simulink model "DCPF_WithDroopCPL"  (R2015b)
settings: Solver=VariableStepAuto  StartTime=0.0  StopTime=1.0  RelTol=1e-3
undefined symbols (not defined in the file or in its folder): C_dc_link, V_dc_link_initial
libraries: powerlib x21
settings Model: Creator=Irina  LastModifiedBy=Irina

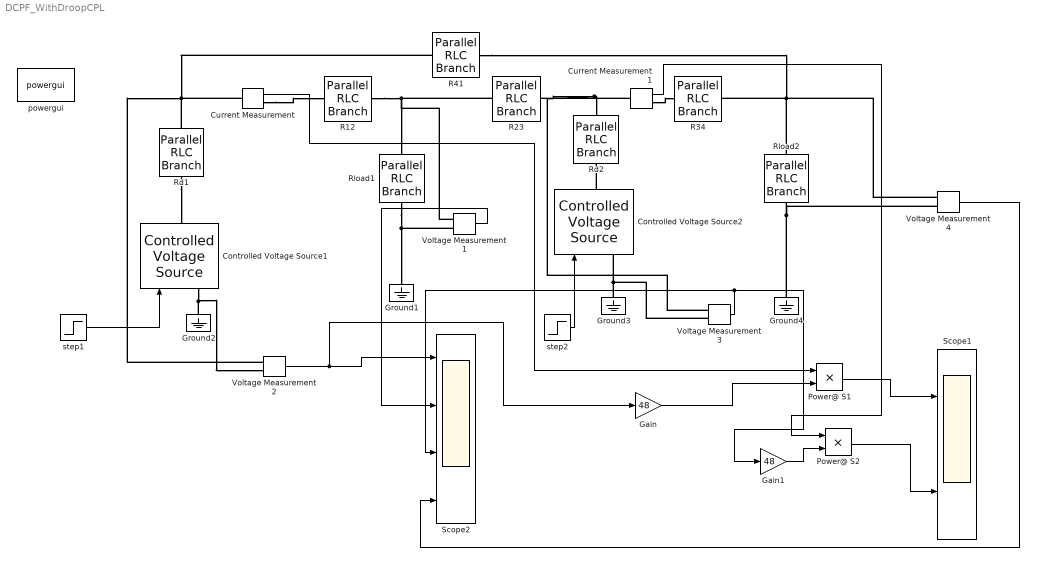
== system DCPF_WithDroopCPL ==
  Controlled Voltage Source1 : powerlib/Electrical Sources/Controlled Voltage Source  Initialize=on  Source_Type=DC  Amplitude=48  Phase=0  Frequency=0  Measurements=None
  Controlled Voltage Source2 : powerlib/Electrical Sources/Controlled Voltage Source  Initialize=on  Source_Type=DC  Amplitude=48  Phase=0  Frequency=0  Measurements=None
  Current Measurement : powerlib/Measurements/Current Measurement  PhasorSimulation=off  OutputType=Complex  PSBequivalent=0
  Current Measurement1 : powerlib/Measurements/Current Measurement  PhasorSimulation=off  OutputType=Complex  PSBequivalent=0
  Gain : Gain  Gain=48
  Gain1 : Gain  Gain=48
  Ground{1..4} (4 alike) : powerlib/Elements/Ground  LConnTagsString=a
  Power@ S1 : Product
  Power@ S2 : Product
  R{12,23,34,41} (4 alike) : powerlib/Elements/Parallel RLC Branch  LConnTagsString=a  RConnTagsString=__new0  BranchType=R  Resistance=0.05  Inductance=1e-3  SetiL0=off  InitialCurrent=0  Capacitance=C_dc_link*2  Setx0=on  InitialVoltage=V_dc_link_initial/2  Measurements=None
  Rd1 : powerlib/Elements/Parallel RLC Branch  LConnTagsString=a  RConnTagsString=__new0  BranchType=R  Resistance=0.2  Inductance=1e-3  SetiL0=off  InitialCurrent=0  Capacitance=C_dc_link*2  Setx0=on  InitialVoltage=V_dc_link_initial/2  Measurements=None
  Rd2 : powerlib/Elements/Parallel RLC Branch  LConnTagsString=a  RConnTagsString=__new0  BranchType=R  Resistance=0.5  Inductance=1e-3  SetiL0=off  InitialCurrent=0  Capacitance=C_dc_link*2  Setx0=on  InitialVoltage=V_dc_link_initial/2  Measurements=None
  Rload1 : powerlib/Elements/Parallel RLC Branch  LConnTagsString=a  RConnTagsString=__new0  BranchType=R  Resistance=9.8  Inductance=1e-3  SetiL0=off  InitialCurrent=0  Capacitance=C_dc_link*2  Setx0=on  InitialVoltage=V_dc_link_initial/2  Measurements=None
  Rload2 : powerlib/Elements/Parallel RLC Branch  LConnTagsString=a  RConnTagsString=__new0  BranchType=R  Resistance=14.54  Inductance=1e-3  SetiL0=off  InitialCurrent=0  Capacitance=C_dc_link*2  Setx0=on  InitialVoltage=V_dc_link_initial/2  Measurements=None
  Scope1 : Scope  NumInputPorts=2
  Scope2 : Scope  NumInputPorts=4
  Voltage Measurement{1..4} (4 alike) : powerlib/Measurements/Voltage Measurement  PhasorSimulation=off  OutputType=Complex  PSBequivalent=0
  powergui : powerlib/powergui  Priority=1  SimulationMode=Discrete  SolverType=Tustin/Backward Euler (TBE)  SampleTime=50e-6  frequency=60  SPID=off  DisableSnubberDevices=off  DisableRonSwitches=off  DisableVfSwitches=off  SwTol=0  DisplayEquations=off  Interpol=off  ExternalGateDelay=off  methode=off  Ts=10  FunctionMessages=off  echomessages=off  HookPort=off  EnableUseOfTLC=off  x0status=blocks  frequencyindice=0  Pbase=100e6  ErrMax=1e-4  Iterations=50  UnitsV=kV  UnitsW=MW  buscounter=0  RestoreLinks=warning  ResistiveCurrentMeasurement=off  Frange=[0:2:500]  Ylog=off  Xlog=on  ShowGrid=off  save=off  variable=ZData  structure=0  ZoomFFT=off  StartTime=0.0  cycles=1  DisplayStyle=1  fundamental=60  FreqAxis=off  MaxFrequency=1000  frequencyindicesteady=1  RmsSteady=1  display=off
  step1 : Step  Time=0.01
  step2 : Step  Time=0.01
  wires:
  Voltage Measurement2/1 -> Gain/1, Scope2/1
  Voltage Measurement1/1 -> Scope2/2
  Voltage Measurement3/1 -> Scope2/3, Gain1/1
  Voltage Measurement4/1 -> Scope2/4
  step1/1 -> Controlled Voltage Source1/1
  step2/1 -> Controlled Voltage Source2/1
  Current Measurement/1 -> Power@ S1/1
  Power@ S1/1 -> Scope1/1
  Current Measurement1/1 -> Power@ S2/1
  Power@ S2/1 -> Scope1/2
  Gain/1 -> Power@ S1/2
  Gain1/1 -> Power@ S2/2
  connections:
  Rd1/LConn1 -- Controlled Voltage Source1/RConn1
  Rd1/RConn1 -- Current Measurement/LConn1 -- Voltage Measurement2/LConn1 -- R41/LConn1
  R12/RConn1 -- Voltage Measurement1/LConn1 -- Rload1/LConn1 -- R23/LConn1
  Rload1/RConn1 -- Ground1/LConn1 -- Voltage Measurement1/LConn2
  Ground3/LConn1 -- Voltage Measurement3/LConn2 -- Controlled Voltage Source2/LConn1
  Voltage Measurement3/LConn1 -- R23/RConn1 -- Current Measurement1/LConn1 -- Rd2/RConn1
  Controlled Voltage Source2/RConn1 -- Rd2/LConn1
  Ground4/LConn1 -- Voltage Measurement4/LConn2 -- Rload2/RConn1
  Rload2/LConn1 -- Voltage Measurement4/LConn1 -- R41/RConn1 -- R34/RConn1
  Ground2/LConn1 -- Voltage Measurement2/LConn2 -- Controlled Voltage Source1/LConn1
  Current Measurement/RConn1 -- R12/LConn1
  Current Measurement1/RConn1 -- R34/LConn1
